simulink model "RRpendulum_fullstatefeedback"  (R2024b)
settings: Solver=VariableStepAuto  StartTime=0.0  StopTime=15  RelTol=1e-7  AbsTol=1e-8
PreLoadFcn:
  | run RRpendulum_FSB_inverted.mlx
undefined symbols (not defined in the file): A_lin_num, b1_num, b2_num, B_lin_num, C_num, g_num, Kd, L, m_num, q1_0, q2_0, Ts, v1_0, v2_0, z0
libraries: simulink x2, sharedTrackingLibrary x1, digtwin_labo_lib x1
settings Model: Creator=u0130154  LastModifiedBy=u0130154
settings SimscapeCC: SimscapeLogType=all

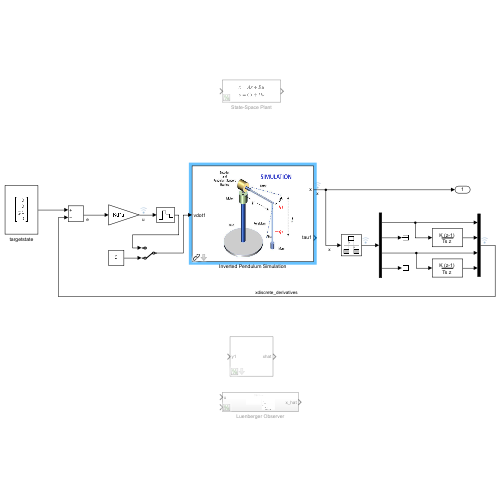
[thumbnail: Simulink's stored preview of the top-level diagram]
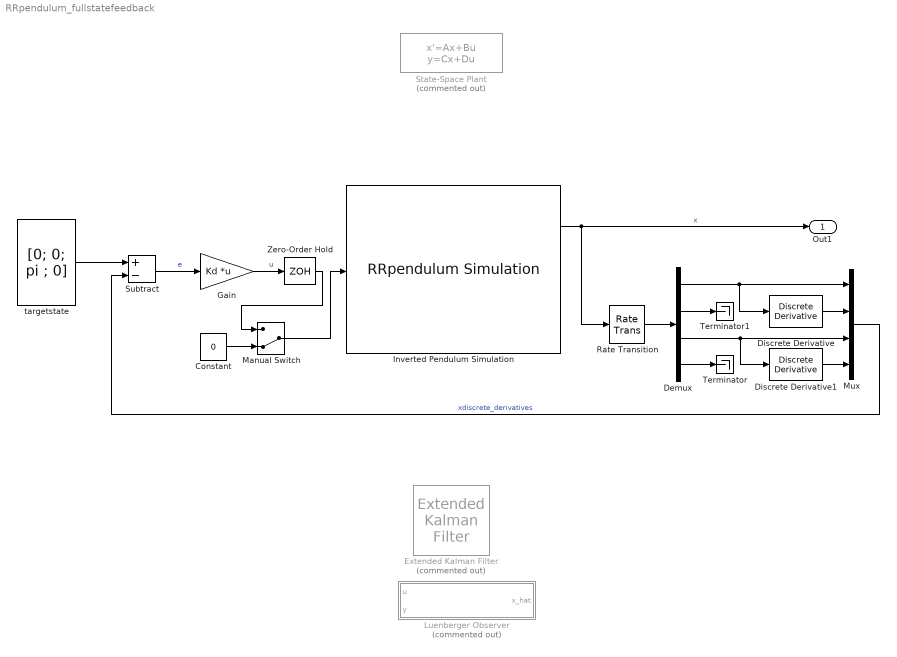
== system RRpendulum_fullstatefeedback ==
  Constant : Constant  Value=0
  Demux : Demux
  Discrete Derivative : simulink/Discrete/Discrete Derivative  gainval=1.0  ICPrevScaledInput=0.0  OutMin=[]  OutMax=[]  OutDataType=fixdt(1, 16)  OutScaling=2^-10  DoSatur=off
  Discrete Derivative1 : simulink/Discrete/Discrete Derivative  gainval=1.0  ICPrevScaledInput=0.0  OutMin=[]  OutMax=[]  OutDataType=fixdt(1, 16)  OutScaling=2^-10  DoSatur=off
  Extended Kalman Filter : sharedTrackingLibrary/Extended Kalman Filter  Commented=on  StateTransitionFcn=myStateTransitionFcn  HasStateTransitionJacobianFcn=off  HasAdditiveProcessNoise=Additive  ProcessNoise=1  HasTimeVaryingProcessNoise=off  HasStateTransitionFcnExtraArgument=0  InitialState=0  InitialStateCovariance=1  MeasurementFcn1=myMeasurementFcn  HasMeasurementJacobianFcn1=off  HasMeasurementEnablePort1=off  HasAdditiveMeasurementNoise1=Additive  MeasurementNoise1=1  HasTimeVaryingMeasurementNoise1=off  HasMeasurementFcnExtraArgument1=0  HasMeasurementWrapping1=off  MeasurementFcn2=myMeasurementFcn  HasMeasurementJacobianFcn2=off  HasMeasurementEnablePort2=off  HasAdditiveMeasurementNoise2=Additive  MeasurementNoise2=1  HasTimeVaryingMeasurementNoise2=off  HasMeasurementFcnExtraArgument2=0  HasMeasurementWrapping2=off  MeasurementFcn3=myMeasurementFcn  HasMeasurementJacobianFcn3=off  HasMeasurementEnablePort3=off  HasAdditiveMeasurementNoise3=Additive  MeasurementNoise3=1  HasTimeVaryingMeasurementNoise3=off  HasMeasurementFcnExtraArgument3=0  HasMeasurementWrapping3=off  MeasurementFcn4=myMeasurementFcn  HasMeasurementJacobianFcn4=off  HasMeasurementEnablePort4=off  HasAdditiveMeasurementNoise4=Additive  MeasurementNoise4=1  HasTimeVaryingMeasurementNoise4=off  HasMeasurementFcnExtraArgument4=0  HasMeasurementWrapping4=off  MeasurementFcn5=myMeasurementFcn  HasMeasurementJacobianFcn5=off  HasMeasurementEnablePort5=off  HasAdditiveMeasurementNoise5=Additive  MeasurementNoise5=1  HasTimeVaryingMeasurementNoise5=off  HasMeasurementFcnExtraArgument5=0  HasMeasurementWrapping5=off  EnableMultirate=off  StateTransitionFcnSampleTime=1  MeasurementFcn1SampleTime=1  MeasurementFcn2SampleTime=1  MeasurementFcn3SampleTime=1  MeasurementFcn4SampleTime=1  MeasurementFcn5SampleTime=1  UseCurrentEstimator=on  OutputStateCovariance=off  DataType=double  SampleTime=1  NumberOfMeasurements=1
  Gain : Gain  Gain=Kd  Multiplication=Matrix(K*u)
  Inverted Pendulum Simulation : digtwin_labo_lib/RRpendulum Simulation  VariantControl=(sim)  initstate=[q1_0; v1_0 ;q2_0; v2_0]  satlimits=satlimits  g=g_num  m=m_num  r=r_num  l=l_num  b=[b1_num b2_num]
  Luenberger Observer : Subsystem  Commented=on
  Manual Switch : ManualSwitch  CurrentSetting=0
  Mux : Mux
  Rate Transition : RateTransition  OutPortSampleTime=Ts
  State-Space Plant : StateSpace  Commented=on  A=A_lin_num  B=B_lin_num  C=eye(4)  D=zeros(4,1)  InitialCondition=z0
  Subtract : Sum  Inputs=+-
  Terminator : Terminator
  Terminator1 : Terminator
  Zero-Order Hold : ZeroOrderHold  SampleTime=Ts
  targetstate : Constant  Value=[0; 0; pi ; 0]  VectorParams1D=off
  Out1 : Outport
  wires:
  Gain/1 -> Zero-Order Hold/1  "u"
  targetstate/1 -> Subtract/1
  Subtract/1 -> Gain/1  "e"
  Rate Transition/1 -> Demux/1
  Inverted Pendulum Simulation/1 -> Out1/1, Rate Transition/1  "x"
  Demux/1 -> Discrete Derivative/1, Mux/1
  Demux/3 -> Discrete Derivative1/1, Mux/3
  Discrete Derivative/1 -> Mux/2
  Discrete Derivative1/1 -> Mux/4
  Demux/2 -> Terminator1/1
  Demux/4 -> Terminator/1
  Mux/1 -> Subtract/2  "xdiscrete_derivatives"
  Constant/1 -> Manual Switch/2
  Manual Switch/1 -> Inverted Pendulum Simulation/1
  Zero-Order Hold/1 -> Manual Switch/1

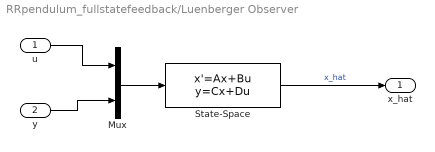
== system RRpendulum_fullstatefeedback/Luenberger Observer ==
  u : Inport
  y : Inport  Port=2
  Mux : Mux  Inputs=2
  State-Space : StateSpace  A=A_lin_num - L*C_num  B=[B_lin_num, L]  C=eye(4)  D=zeros(4,3)  InitialCondition=z0
  x_hat : Outport
  wires:
  Mux/1 -> State-Space/1
  u/1 -> Mux/1
  y/1 -> Mux/2
  State-Space/1 -> x_hat/1  "x_hat"
